simulink model "smm_with_grf_tilting_2d"  (R2014b)
settings: Solver=FixedStepDiscrete  StartTime=0.0  StopTime=inf  FixedStep=sample_time  RelTol=1e-3
undefined symbols (not defined in the file or in its folder): A_kalman_fourbar_gear, A_kalman_transverse, A_kalman_vertical, A_lpf_dtau, A_lpf_leg_spring, alpha_apex, B1_lpf_dtau, B1_lpf_leg_spring, B2_lpf_dtau, B2_lpf_leg_spring, B_kalman_fourbar_gear, B_kalman_transverse, B_kalman_vertical, b_virtual, boom_mount_angle, c_energy, C_kalman_fourbar_gear, C_kalman_transverse, C_kalman_vertical, com_leg_motor, com_torso, contact_threshold, control_start_time, d_vertical_boom_com_offset, d_vertical_com, d_y_com, desired_com_apex_height, desired_com_forward_velocity, desired_torso_angle, Discrete, fcut_contact, g, h_boom, HIP_MTR_MAX_CONT_TORQUE, i_robot, initial_dx_estimate, initial_dy_estimate, initial_dz_estimate, initial_z_estimate, j_leg, j_motor, j_rotor, j_segments, k0_virtual, k_placement, k_sea, kalman_load_to_deflect_transmission, kalman_stance_slip_threshold, kd_lateral, kd_motor, kd_torso, kp_lateral, kp_motor, kp_torso, l0_leg, l0_virtual, l_boom_projected, l_retract_delta, l_retract_swing_max, l_retract_swing_min ... (+59)
libraries: simulink x25, ctrlSharedLib x7, simulink_extras x1
(part 2 of 4)

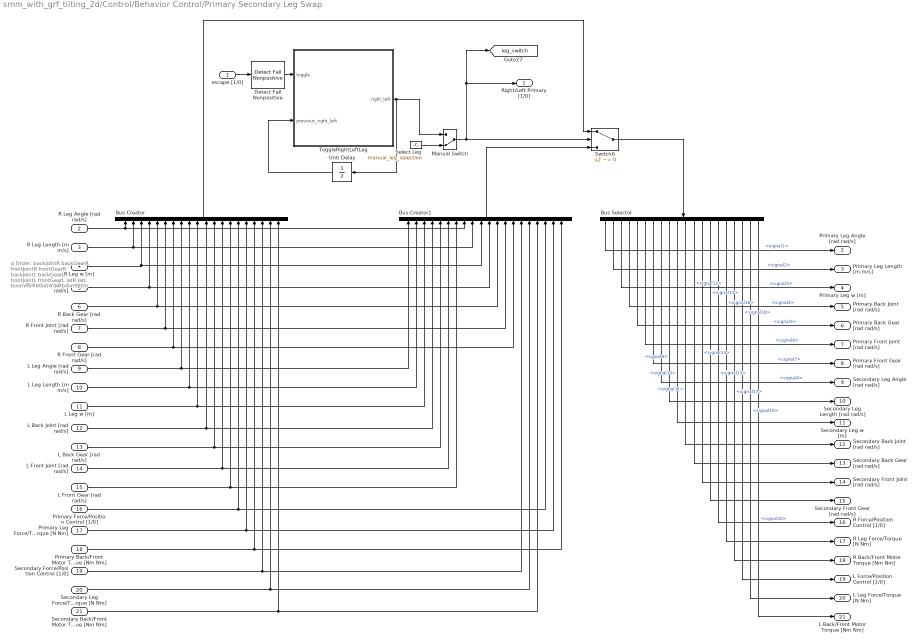
== system smm_with_grf_tilting_2d/Control/Behavior Control/Primary Secondary Leg Swap ==
  note: q Order:
      |
      | backJointR
      | backGearR
      | frontJointR
      | frontGearR
      |
      | backJointL
      | backGearL
      | frontJointL
      | frontGearL
      |
      | latR
      | latL
      |
      | boomRoll
      | boomYaw
      | boomPitch
  escape [1/0] : Inport
  R Leg Angle [rad rad/s] : Inport  Port=2
  R Leg Length [m m/s] : Inport  Port=3
  R Leg w [m] : Inport  Port=4
  R Back Joint [rad rad/s] : Inport  Port=5
  R Back Gear [rad rad/s] : Inport  Port=6
  R Front Joint [rad rad/s] : Inport  Port=7
  R Front Gear [rad rad/s] : Inport  Port=8
  L Leg Angle [rad rad/s] : Inport  Port=9
  L Leg Length [m m/s] : Inport  Port=10
  L Leg w [m] : Inport  Port=11
  L Back Joint [rad rad/s] : Inport  Port=12
  L Back Gear [rad rad/s] : Inport  Port=13
  L Front Joint [rad rad/s] : Inport  Port=14
  L Front Gear [rad rad/s] : Inport  Port=15
  Primary Force/Position Control [1/0] : Inport  Port=16
  Primary Leg Force/Torque [N Nm] : Inport  Port=17
  Primary Back/Front Motor Torque [Nm Nm] : Inport  Port=18
  Secondary Force/Position Control [1/0] : Inport  Port=19
  Secondary Leg Force/Torque [N Nm] : Inport  Port=20
  Secondary Back/Front Motor Torque [Nm Nm] : Inport  Port=21
  Bus Creator : BusCreator  Inputs=20
  Bus Creator1 : BusCreator  Inputs=20
  Bus Selector : BusSelector  OutputSignals=signal1,signal2,signal3,signal4,signal5,signal6,signal7,signal8,signal9,signal10,signal11,signal12,signal13,signal14,signal15,signal16,signal17,signal18,signal19,signal20
  Detect Fall Nonpositive : simulink/Logic and Bit Operations/Detect Fall Nonpositive  vinit=0  InputProcessing=Inherited  OutDataTypeStr=boolean
  Manual Switch : ManualSwitch  CurrentSetting=0
  Select Leg : Constant  Value=manual_leg_selection  OutDataTypeStr=boolean
  Switch6 : Switch  Criteria=u2 ~= 0  OutDataTypeStr=Inherit: Inherit via back propagation  ZeroCross=off
  ToggleRightLeftLeg : MATLAB Function  TreatAsAtomicUnit=on
      settings: MinAlgLoopOccurrences=on
  Unit Delay : UnitDelay  InitialCondition=1  SampleTime=sample_time
  Right/Left Primary [1/0] : Outport
  Primary Leg Angle [rad rad/s] : Outport  Port=2
  Primary Leg Length [m m/s] : Outport  Port=3
  Primary Leg w [m] : Outport  Port=4
  Primary Back Joint [rad rad/s] : Outport  Port=5
  Primary Back Gear [rad rad/s] : Outport  Port=6
  Primary Front Joint [rad rad/s] : Outport  Port=7
  Primary Front Gear [rad rad/s] : Outport  Port=8
  Secondary Leg Angle [rad rad/s] : Outport  Port=9
  Secondary Leg Length [rad rad/s] : Outport  Port=10
  Secondary Leg w [m] : Outport  Port=11
  Secondary Back Joint [rad rad/s] : Outport  Port=12
  Secondary Back Gear [rad rad/s] : Outport  Port=13
  Secondary Front Joint [rad rad/s] : Outport  Port=14
  Secondary Front Gear [rad rad/s] : Outport  Port=15
  R Force/Position Control [1/0] : Outport  Port=16
  R Leg Force/Torque [N Nm] : Outport  Port=17
  R Back/Front Motor Torque [Nm Nm] : Outport  Port=18
  L Force/Position Control [1/0] : Outport  Port=19
  L Leg Force/Torque [N Nm] : Outport  Port=20
  L Back/Front Motor Torque [Nm Nm] : Outport  Port=21
  tag scope: leg_switch=global
  wires:
  Unit Delay/1 -> ToggleRightLeftLeg/2(previous_right_left)
  Detect Fall Nonpositive/1 -> ToggleRightLeftLeg/1(toggle)
  escape [1/0]/1 -> Detect Fall Nonpositive/1
  ToggleRightLeftLeg/1(right_left) -> Unit Delay/1, Manual Switch/1
  Manual Switch/1 -> [leg_switch], Right/Left Primary [1/0]/1, Switch6/2
  Select Leg/1 -> Manual Switch/2
  R Leg w [m]/1 -> Bus Creator1/10, Bus Creator/3
  R Leg Angle [rad rad/s]/1 -> Bus Creator1/8, Bus Creator/1
  R Leg Length [m m/s]/1 -> Bus Creator1/9, Bus Creator/2
  Bus Creator/1 -> Switch6/1
  Bus Creator1/1 -> Switch6/3
  R Back Joint [rad rad/s]/1 -> Bus Creator1/11, Bus Creator/4
  R Back Gear [rad rad/s]/1 -> Bus Creator1/12, Bus Creator/5
  R Front Joint [rad rad/s]/1 -> Bus Creator1/13, Bus Creator/6
  R Front Gear [rad rad/s]/1 -> Bus Creator1/14, Bus Creator/7
  L Leg Angle [rad rad/s]/1 -> Bus Creator1/1, Bus Creator/8
  L Leg Length [m m/s]/1 -> Bus Creator1/2, Bus Creator/9
  L Leg w [m]/1 -> Bus Creator1/3, Bus Creator/10
  L Back Joint [rad rad/s]/1 -> Bus Creator1/4, Bus Creator/11
  L Back Gear [rad rad/s]/1 -> Bus Creator1/5, Bus Creator/12
  L Front Joint [rad rad/s]/1 -> Bus Creator/13, Bus Creator1/6
  L Front Gear [rad rad/s]/1 -> Bus Creator1/7, Bus Creator/14
  Primary Force/Position Control [1/0]/1 -> Bus Creator1/18, Bus Creator/15
  Primary Leg Force/Torque [N Nm]/1 -> Bus Creator1/19, Bus Creator/16
  Primary Back/Front Motor Torque [Nm Nm]/1 -> Bus Creator1/20, Bus Creator/17
  Secondary Force/Position Control [1/0]/1 -> Bus Creator1/15, Bus Creator/18
  Secondary Leg Force/Torque [N Nm]/1 -> Bus Creator1/16, Bus Creator/19
  Secondary Back/Front Motor Torque [Nm Nm]/1 -> Bus Creator1/17, Bus Creator/20
  Switch6/1 -> Bus Selector/1
  Bus Selector/1 -> Primary Leg Angle [rad rad/s]/1  "<signal1>"
  Bus Selector/2 -> Primary Leg Length [m m/s]/1  "<signal2>"
  Bus Selector/3 -> Primary Leg w [m]/1  "<signal3>"
  Bus Selector/4 -> Primary Back Joint [rad rad/s]/1  "<signal4>"
  Bus Selector/5 -> Primary Back Gear [rad rad/s]/1  "<signal5>"
  Bus Selector/6 -> Primary Front Joint [rad rad/s]/1  "<signal6>"
  Bus Selector/7 -> Primary Front Gear [rad rad/s]/1  "<signal7>"
  Bus Selector/8 -> Secondary Leg Angle [rad rad/s]/1  "<signal8>"
  Bus Selector/9 -> Secondary Leg Length [rad rad/s]/1  "<signal9>"
  Bus Selector/10 -> Secondary Leg w [m]/1  "<signal10>"
  Bus Selector/11 -> Secondary Back Joint [rad rad/s]/1  "<signal11>"
  Bus Selector/12 -> Secondary Back Gear [rad rad/s]/1  "<signal12>"
  Bus Selector/13 -> Secondary Front Joint [rad rad/s]/1  "<signal13>"
  Bus Selector/14 -> Secondary Front Gear [rad rad/s]/1  "<signal14>"
  Bus Selector/15 -> R Force/Position Control [1/0]/1  "<signal15>"
  Bus Selector/16 -> R Leg Force/Torque [N Nm]/1  "<signal16>"
  Bus Selector/17 -> R Back/Front Motor Torque [Nm Nm]/1  "<signal17>"
  Bus Selector/18 -> L Force/Position Control [1/0]/1  "<signal18>"
  Bus Selector/19 -> L Leg Force/Torque [N Nm]/1  "<signal19>"
  Bus Selector/20 -> L Back/Front Motor Torque [Nm Nm]/1  "<signal20>"

== system smm_with_grf_tilting_2d/Control/Behavior Control/R Leg Calculator ==
  Front [rad rad/s] : Inport
  Back [rad rad/s] : Inport  Port=2
  Demux1 : Demux  Outputs=2
  Gain1 : Gain  Gain=2*l_seg
  Gain2 : Gain  Gain=l_seg
  Gain3 : Gain  Gain=-1
  Gain4 : Gain  Gain=0.5
  Gain5 : Gain  Gain=0.5
  Gain6 : Gain  Gain=2
  Mux1 : Mux  Inputs=2
  Product : Product  RndMeth=Zero
  Sum4 : Sum  Inputs=+|+
  Sum5 : Sum  Inputs=+|-
  Trigonometric Function : Trigonometry  Operator=cos
  Trigonometric Function1 : Trigonometry
  "Leg Length [m m/s] " : Outport
  Leg Angle [rad rad/s] : Outport  Port=2
  Leg Splay [rad rad/s] : Outport  Port=3
  w [m] : Outport  Port=4
  wires:
  Gain5/1 -> Leg Angle [rad rad/s]/1
  Sum4/1 -> Gain5/1
  Mux1/1 -> "Leg Length [m m/s] "/1
  Sum5/1 -> Demux1/1, Leg Splay [rad rad/s]/1
  Gain2/1 -> Gain6/1, Product/1
  Demux1/1 -> Gain4/1
  Gain3/1 -> Product/2
  Demux1/2 -> Gain3/1
  Back [rad rad/s]/1 -> Sum5/1, Sum4/1
  Front [rad rad/s]/1 -> Sum4/2, Sum5/2
  Product/1 -> Mux1/2
  Trigonometric Function1/1 -> Gain2/1
  Gain1/1 -> Mux1/1
  Trigonometric Function/1 -> Gain1/1
  Gain4/1 -> Trigonometric Function/1, Trigonometric Function1/1
  Gain6/1 -> w [m]/1

== system smm_with_grf_tilting_2d/Control/Behavior Control/Raibert Initiated ==
  Enable : EnablePort  StatesWhenEnabling=reset
  Constant : Constant
  Hopping? : Outport  InitialOutput=[0]
  wires:
  Constant/1 -> Hopping?/1

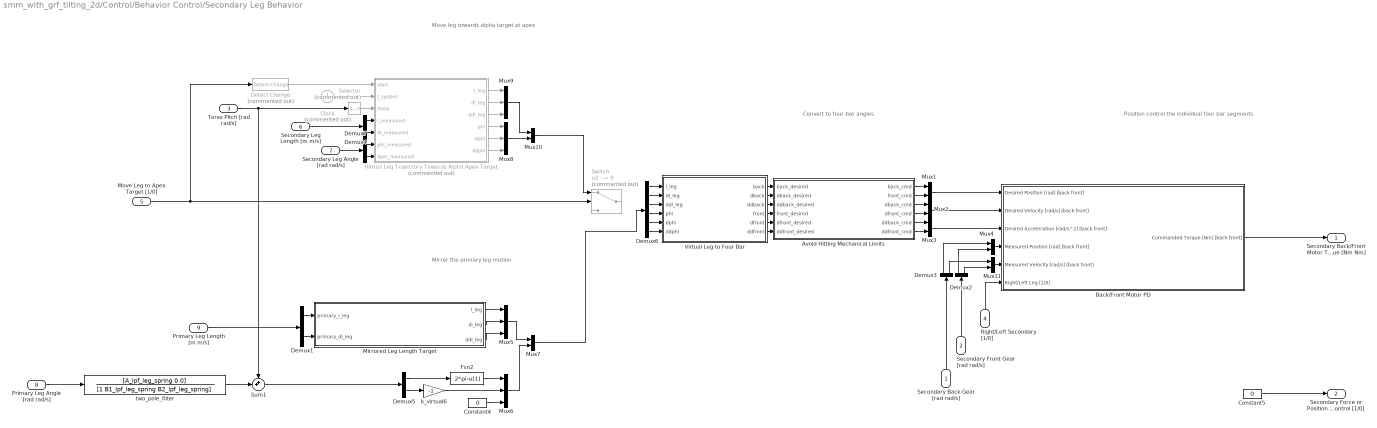
== system smm_with_grf_tilting_2d/Control/Behavior Control/Secondary Leg Behavior ==
  note: Mirror the primary
      | leg motion
  note: Move leg towards
      | alpha target at apex
  note: Position control the
      | individual four bar segments
  note: Convert to
      | four-bar angles
  Secondary Back Gear [rad rad/s] : Inport
  Secondary Front Gear [rad rad/s] : Inport  Port=2
  Torso Pitch [rad rad/s] : Inport  Port=3
  Right/Left Secondary [1/0] : Inport  Port=4
  Move Leg to Apex Target [1/0] : Inport  Port=5
  Secondary Leg Length [m m/s] : Inport  Port=6
  Secondary Leg Angle [rad rad/s] : Inport  Port=7
  Primary Leg Angle [rad rad/s] : Inport  Port=8
  Primary Leg Length [m m/s] : Inport  Port=9
  Avoid Hitting Mechanical Limits : MATLAB Function  TreatAsAtomicUnit=on
  Back/Front Motor PD : Subsystem
  Clock : Clock  Commented=on
  Constant4 : Constant  Value=0
  Constant5 : Constant  Value=0  OutDataTypeStr=boolean
  Demux{1..5,7} (6 alike) : Demux  Outputs=2
  Demux6 : Demux  Outputs=6
  Detect Change : simulink/Logic and Bit Operations/Detect Change  Commented=on  vinit=0  InputProcessing=Inherited  OutDataTypeStr=boolean
  Fcn2 : Fcn  Expr=2*pi-u(1)
  Mirrored Leg Length Target : MATLAB Function  TreatAsAtomicUnit=on
  Mux{1..4,7,10..11} (7 alike) : Mux  Inputs=2
  Mux{5..6,8..9} (4 alike) : Mux  Inputs=3
  Selector : Selector  Commented=on  InputPortWidth=2  Indices=[1]
  Sum1 : Sum  Inputs=++|
  Switch : Switch  Commented=on  Criteria=u2 ~= 0
  Virtual Leg Trajectory Towards Alpha Apex Target : MATLAB Function  Commented=on  TreatAsAtomicUnit=on
  Virtual Leg to Four Bar : MATLAB Function  TreatAsAtomicUnit=on
  k_virtual6 : Gain  Gain=-1
  two_pole_filter : DiscreteTransferFcn  Numerator=[A_lpf_leg_spring 0 0]  Denominator=[1 B1_lpf_leg_spring B2_lpf_leg_spring]  SampleTime=sample_time
  Secondary Back/Front Motor Torque [Nm Nm] : Outport
  Secondary Force or Position Control [1/0] : Outport  Port=2
  wires:
  Constant5/1 -> Secondary Force or Position Control [1/0]/1
  Back/Front Motor PD/1(Commanded Torque [Nm] [back front]) -> Secondary Back/Front Motor Torque [Nm Nm]/1
  Demux5/2 -> k_virtual6/1
  Demux5/1 -> Fcn2/1
  Primary Leg Angle [rad rad/s]/1 -> two_pole_filter/1
  Mirrored Leg Length Target/2(dl_leg) -> Mux5/2
  Mirrored Leg Length Target/3(ddl_leg) -> Mux5/3
  Mirrored Leg Length Target/1(l_leg) -> Mux5/1
  Constant4/1 -> Mux6/3
  k_virtual6/1 -> Mux6/2
  Fcn2/1 -> Mux6/1
  Move Leg to Apex Target [1/0]/1 -> Detect Change/1, Switch/2
  Mux7/1 -> Demux6/1
  Mux9/1 -> Mux10/1
  Mux8/1 -> Mux10/2
  Mux10/1 -> Switch/1
  Torso Pitch [rad rad/s]/1 -> Selector/1, Sum1/1
  Selector/1 -> Virtual Leg Trajectory Towards Alpha Apex Target/3(theta)
  Mux5/1 -> Mux7/1
  Mux6/1 -> Mux7/2
  Virtual Leg Trajectory Towards Alpha Apex Target/6(ddphi) -> Mux8/3
  Virtual Leg Trajectory Towards Alpha Apex Target/5(dphi) -> Mux8/2
  Virtual Leg Trajectory Towards Alpha Apex Target/4(phi) -> Mux8/1
  Virtual Leg Trajectory Towards Alpha Apex Target/3(ddl_leg) -> Mux9/3
  Virtual Leg Trajectory Towards Alpha Apex Target/2(dl_leg) -> Mux9/2
  Virtual Leg Trajectory Towards Alpha Apex Target/1(l_leg) -> Mux9/1
  Detect Change/1 -> Virtual Leg Trajectory Towards Alpha Apex Target/1(start)
  Clock/1 -> Virtual Leg Trajectory Towards Alpha Apex Target/2(t_system)
  Demux4/2 -> Virtual Leg Trajectory Towards Alpha Apex Target/5(dl_measured)
  Demux4/1 -> Virtual Leg Trajectory Towards Alpha Apex Target/4(l_measured)
  Demux7/1 -> Virtual Leg Trajectory Towards Alpha Apex Target/6(phi_measured)
  Demux7/2 -> Virtual Leg Trajectory Towards Alpha Apex Target/7(dphi_measured)
  Secondary Leg Length [m m/s]/1 -> Demux4/1
  Secondary Leg Angle [rad rad/s]/1 -> Demux7/1
  Virtual Leg to Four Bar/1(back) -> Avoid Hitting Mechanical Limits/1(back_desired)
  Virtual Leg to Four Bar/2(dback) -> Avoid Hitting Mechanical Limits/2(dback_desired)
  Virtual Leg to Four Bar/3(ddback) -> Avoid Hitting Mechanical Limits/3(ddback_desired)
  Virtual Leg to Four Bar/4(front) -> Avoid Hitting Mechanical Limits/4(front_desired)
  Virtual Leg to Four Bar/5(dfront) -> Avoid Hitting Mechanical Limits/5(dfront_desired)
  Virtual Leg to Four Bar/6(ddfront) -> Avoid Hitting Mechanical Limits/6(ddfront_desired)
  Demux6/1 -> Virtual Leg to Four Bar/1(l_leg)
  Demux6/2 -> Virtual Leg to Four Bar/2(dl_leg)
  Demux6/3 -> Virtual Leg to Four Bar/3(ddl_leg)
  Demux6/4 -> Virtual Leg to Four Bar/4(phi)
  Demux6/5 -> Virtual Leg to Four Bar/5(dphi)
  Demux6/6 -> Virtual Leg to Four Bar/6(ddphi)
  Mux11/1 -> Back/Front Motor PD/5(Measured Velocity [rad/s] [back front])
  Demux2/2 -> Mux11/2
  Mux4/1 -> Back/Front Motor PD/4(Measured Position [rad] [back front])
  Mux1/1 -> Back/Front Motor PD/1(Desired Position [rad] [back front])
  Right/Left Secondary [1/0]/1 -> Back/Front Motor PD/6(Right/Left Leg [1/0])
  Demux3/2 -> Mux11/1
  Demux3/1 -> Mux4/1
  Avoid Hitting Mechanical Limits/2(front_cmd) -> Mux1/2
  Avoid Hitting Mechanical Limits/1(back_cmd) -> Mux1/1
  Demux2/1 -> Mux4/2
  Secondary Front Gear [rad rad/s]/1 -> Demux2/1
  Secondary Back Gear [rad rad/s]/1 -> Demux3/1
  Avoid Hitting Mechanical Limits/3(dback_cmd) -> Mux2/1
  Avoid Hitting Mechanical Limits/4(dfront_cmd) -> Mux2/2
  Avoid Hitting Mechanical Limits/5(ddback_cmd) -> Mux3/1
  Avoid Hitting Mechanical Limits/6(ddfront_cmd) -> Mux3/2
  Mux2/1 -> Back/Front Motor PD/2(Desired Velocity [rad/s] [back front])
  Mux3/1 -> Back/Front Motor PD/3(Desired Acceleration [rad/s^2] [back front])
  two_pole_filter/1 -> Sum1/2
  Sum1/1 -> Demux5/1
  Demux1/1 -> Mirrored Leg Length Target/1(primary_l_leg)
  Demux1/2 -> Mirrored Leg Length Target/2(primary_dl_leg)
  Primary Leg Length [m m/s]/1 -> Demux1/1

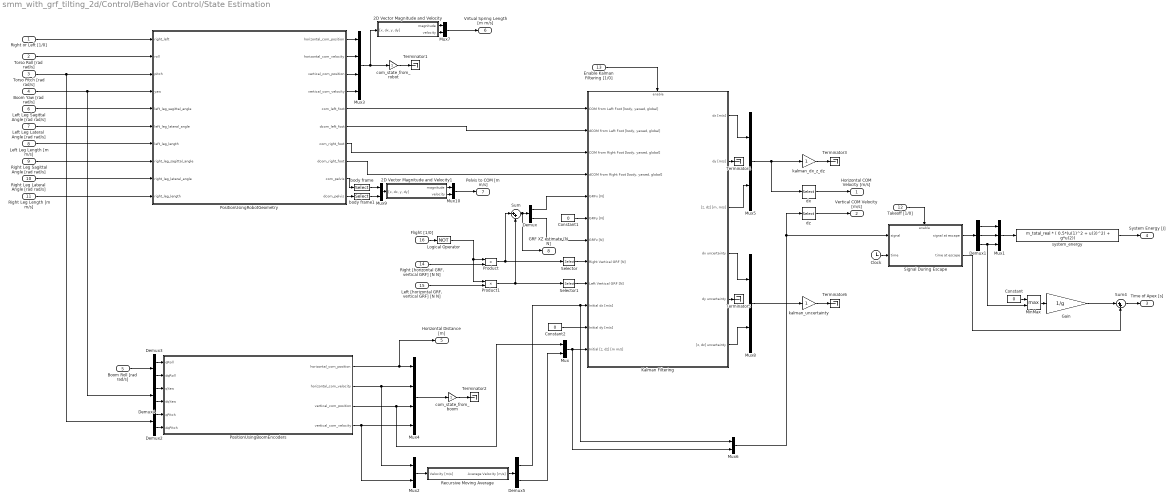
== system smm_with_grf_tilting_2d/Control/Behavior Control/State Estimation ==
  Right or Left [1/0] : Inport
  Torso Roll [rad rad/s] : Inport  Port=2
  Torso Pitch [rad rad/s] : Inport  Port=3
  Boom Yaw [rad rad/s] : Inport  Port=4
  Boom Roll [rad rad/s] : Inport  Port=5
  Left Leg Sagittal Angle [rad rad/s] : Inport  Port=6
  Left Leg Lateral  Angle [rad rad/s] : Inport  Port=7
  Left Leg Length [m m/s] : Inport  Port=8
  Right Leg Sagittal Angle [rad rad/s] : Inport  Port=9
  Right Leg Lateral  Angle [rad rad/s] : Inport  Port=10
  Right Leg Length [m m/s] : Inport  Port=11
  Takeoff [1/0] : Inport  Port=12
  Enable Kalman Filtering [1/0] : Inport  Port=13
  "Right [horizontal GRF, vertical GRF] [N N]" : Inport  Port=14
  "Left [horizontal GRF, vertical GRF] [N N]" : Inport  Port=15
  Flight [1/0] : Inport  Port=16
  2D Vector Magnitude and Velocity : Subsystem
  2D Vector Magnitude and Velocity1 : Subsystem
  Clock : Clock
  Constant : Constant  Value=0
  Constant1 : Constant  Value=0
  Constant2 : Constant  Value=0
  Demux{,2..5} (5 alike) : Demux  Outputs=2
  Demux1 : Demux  Outputs=3
  Gain : Gain  Gain=1/g
  Kalman Filtering : Subsystem
  Logical Operator : Logic  Operator=NOT  AllPortsSameDT=off  OutDataTypeStr=boolean
  MinMax : MinMax  Function=max  Inputs=2
  Mux{,2,5..10} (8 alike) : Mux  Inputs=2
  Mux1 : Mux  Inputs=3
  Mux3 : Mux
  Mux4 : Mux
  PositionUsingBoomEncoders : MATLAB Function  TreatAsAtomicUnit=on
  PositionUsingRobotGeometry : MATLAB Function  TreatAsAtomicUnit=on
  Product : Product
  Product1 : Product
  Recursive Moving Average : Subsystem
  Selector : Selector  InputPortWidth=2  Indices=[2]
  Selector1 : Selector  InputPortWidth=2  Indices=[2]
  Signal During Escape : Subsystem
  Sum : Sum  Inputs=|++
  Sum4 : Sum  Inputs=|++
  Terminator{1..6} (6 alike) : Terminator
  body frame : Selector  InputPortWidth=9  Indices=[1 3]
  body frame1 : Selector  InputPortWidth=9  Indices=[1 3]
  com_state_from_boom : Gain
  com_state_from_robot : Gain
  dx : Selector  InputPortWidth=3  Indices=[1]
  dz : Selector  InputPortWidth=3  Indices=[3]
  kalman_dx_z_dz : Gain
  kalman_uncertainty : Gain
  system_energy : Fcn  Expr=m_total_real * ( 0.5*(u(1)^2 + u(3)^2) + g*u(2))
  Horizontal COM Velocity [m/s] : Outport
  Vertical COM Velocity [m/s] : Outport  Port=2
  Time of Apex [s] : Outport  Port=3
  System Energy [J] : Outport  Port=4
  Horizontal Distance [m] : Outport  Port=5
  Virtual Spring Length [m m/s] : Outport  Port=6
  Pelvis to COM [m m/s] : Outport  Port=7
  GRF XZ estimate [N N] : Outport  Port=8
  wires:
  Gain/1 -> Sum4/1
  com_state_from_boom/1 -> Terminator2/1
  system_energy/1 -> System Energy [J]/1
  Clock/1 -> Signal During Escape/2(time)
  Demux1/3 -> MinMax/2, Mux1/3
  Signal During Escape/2(time at escape) -> Sum4/2
  Takeoff [1/0]/1 -> Signal During Escape/Enable
  Mux1/1 -> system_energy/1
  Demux1/1 -> Mux1/1
  Demux1/2 -> Mux1/2
  Sum4/1 -> Time of Apex [s]/1
  Kalman Filtering/1(dx [m/s]) -> Mux5/1
  MinMax/1 -> Gain/1
  Constant/1 -> MinMax/1
  Demux2/1 -> PositionUsingBoomEncoders/5(qPitch)
  Demux2/2 -> PositionUsingBoomEncoders/6(dqPitch)
  Mux3/1 -> 2D Vector Magnitude and Velocity/1("[x, dx, y, dy]"), com_state_from_robot/1
  com_state_from_robot/1 -> Terminator1/1
  PositionUsingRobotGeometry/4(vertical_com_velocity) -> Mux3/4
  PositionUsingRobotGeometry/3(vertical_com_position) -> Mux3/3
  PositionUsingRobotGeometry/2(horizontal_com_velocity) -> Mux3/2
  PositionUsingRobotGeometry/1(horizontal_com_position) -> Mux3/1
  PositionUsingBoomEncoders/1(horizontal_com_position) -> Horizontal Distance [m]/1, Mux4/1
  PositionUsingBoomEncoders/3(vertical_com_position) -> Mux/1, Mux4/3
  PositionUsingBoomEncoders/4(vertical_com_velocity) -> Mux2/2, Mux4/4
  Mux4/1 -> com_state_from_boom/1
  Left Leg Sagittal Angle [rad rad/s]/1 -> PositionUsingRobotGeometry/5(left_leg_sagittal_angle)
  Left Leg Lateral  Angle [rad rad/s]/1 -> PositionUsingRobotGeometry/6(left_leg_lateral_angle)
  Left Leg Length [m m/s]/1 -> PositionUsingRobotGeometry/7(left_leg_length)
  Right Leg Sagittal Angle [rad rad/s]/1 -> PositionUsingRobotGeometry/8(right_leg_sagittal_angle)
  Right Leg Lateral  Angle [rad rad/s]/1 -> PositionUsingRobotGeometry/9(right_leg_lateral_angle)
  Right Leg Length [m m/s]/1 -> PositionUsingRobotGeometry/10(right_leg_length)
  Right or Left [1/0]/1 -> PositionUsingRobotGeometry/1(right_left)
  Torso Roll [rad rad/s]/1 -> PositionUsingRobotGeometry/2(roll)
  Boom Yaw [rad rad/s]/1 -> PositionUsingRobotGeometry/4(yaw), Demux4/1
  Torso Pitch [rad rad/s]/1 -> PositionUsingRobotGeometry/3(pitch), Demux2/1
  Demux3/2 -> PositionUsingBoomEncoders/2(dqRoll)
  Demux3/1 -> PositionUsingBoomEncoders/1(qRoll)
  Boom Roll [rad rad/s]/1 -> Demux3/1
  Demux4/1 -> PositionUsingBoomEncoders/3(qYaw)
  Demux4/2 -> PositionUsingBoomEncoders/4(dqYaw)
  PositionUsingRobotGeometry/5(com_left_foot) -> Kalman Filtering/1("COM from Left Foot [body, yawed, global]")
  PositionUsingRobotGeometry/6(dcom_left_foot) -> Kalman Filtering/2("dCOM from Left Foot [body, yawed, global]")
  PositionUsingRobotGeometry/7(com_right_foot) -> Kalman Filtering/3("COM from Right Foot [body, yawed, global]")
  PositionUsingRobotGeometry/8(dcom_right_foot) -> Kalman Filtering/4("dCOM from Right Foot [body, yawed, global]")
  Kalman Filtering/2(dy [m/s]) -> Terminator4/1
  Kalman Filtering/3("[z, dz] [m, m/s]") -> Mux5/2
  Signal During Escape/1(signal at escape) -> Demux1/1
  Mux2/1 -> Recursive Moving Average/1(Velocity [m/s])
  dx/1 -> Horizontal COM Velocity [m/s]/1
  Mux6/1 -> Signal During Escape/1(signal), dz/1
  dz/1 -> Vertical COM Velocity [m/s]/1
  Constant1/1 -> Kalman Filtering/6(GRFy [N])
  Recursive Moving Average/1(Average Velocity [m/s]) -> Demux5/1
  Mux/1 -> Mux6/2, Kalman Filtering/12("Initial [z, dz] [m m/s]")
  Demux5/2 -> Mux/2
  Constant2/1 -> Kalman Filtering/11(Initial dy [m/s])
  PositionUsingBoomEncoders/2(horizontal_com_velocity) -> Mux2/1, Mux4/2
  Selector/1 -> Kalman Filtering/8(Right Vertical GRF [N])
  Selector1/1 -> Kalman Filtering/9(Left Vertical GRF [N])
  Product1/1 -> Sum/2, Selector1/1
  Product/1 -> Sum/1, Selector/1
  Sum/1 -> GRF XZ estimate [N N]/1, Demux/1
  Enable Kalman Filtering [1/0]/1 -> Kalman Filtering/Enable
  kalman_dx_z_dz/1 -> Terminator3/1
  Mux5/1 -> dx/1, kalman_dx_z_dz/1
  Demux5/1 -> Mux6/1, Kalman Filtering/10(Initial dx [m/s])
  Mux7/1 -> Virtual Spring Length [m m/s]/1
  Demux/1 -> Kalman Filtering/5(GRFx [N])
  Demux/2 -> Kalman Filtering/7(GRFz [N])
  Flight [1/0]/1 -> Logical Operator/1
  "Right [horizontal GRF, vertical GRF] [N N]"/1 -> Product/2
  Logical Operator/1 -> Product1/1, Product/1
  "Left [horizontal GRF, vertical GRF] [N N]"/1 -> Product1/2
  Kalman Filtering/4(dx uncertainty) -> Mux8/1
  Kalman Filtering/6("[z, dz] uncertainty") -> Mux8/2
  Kalman Filtering/5(dy uncertainty) -> Terminator5/1
  kalman_uncertainty/1 -> Terminator6/1
  Mux8/1 -> kalman_uncertainty/1
  PositionUsingRobotGeometry/10(dcom_pelvis) -> body frame1/1
  PositionUsingRobotGeometry/9(com_pelvis) -> body frame/1
  body frame/1 -> Mux9/1
  body frame1/1 -> Mux9/2
  Mux9/1 -> 2D Vector Magnitude and Velocity1/1("[x, dx, y, dy]")
  2D Vector Magnitude and Velocity/1(magnitude) -> Mux7/1
  2D Vector Magnitude and Velocity/2(velocity) -> Mux7/2
  2D Vector Magnitude and Velocity1/1(magnitude) -> Mux10/1
  2D Vector Magnitude and Velocity1/2(velocity) -> Mux10/2
  Mux10/1 -> Pelvis to COM [m m/s]/1

== system smm_with_grf_tilting_2d/Control/Behavior Control/Torque Distribution Left ==
  Leg Torque [Nm] : Inport
  Leg Force [N] : Inport  Port=2
  w [m] : Inport  Port=3
  Gain : Gain  Gain=0.5
  Gain1 : Gain  Gain=0.5
  Motor Torque Saturation Optimization : MATLAB Function  TreatAsAtomicUnit=on
  Product : Product  RndMeth=Zero
  Sum : Sum  Inputs=|++
  Sum1 : Sum  Inputs=+-|
  Back Torque [Nm] : Outport
  Front Torque [Nm] : Outport  Port=2
  wires:
  Gain/1 -> Motor Torque Saturation Optimization/1(x1s)
  Gain1/1 -> Motor Torque Saturation Optimization/2(x2s)
  Product/1 -> Gain1/1
  Leg Force [N]/1 -> Product/1
  Motor Torque Saturation Optimization/2(t2) -> Sum/2, Sum1/2
  w [m]/1 -> Product/2
  Motor Torque Saturation Optimization/1(t1) -> Sum1/1, Sum/1
  Sum/1 -> Front Torque [Nm]/1
  Leg Torque [Nm]/1 -> Gain/1
  Sum1/1 -> Back Torque [Nm]/1

== system smm_with_grf_tilting_2d/Control/Behavior Control/Torque Distribution Right ==
  Leg Torque [Nm] : Inport
  Leg Force [N] : Inport  Port=2
  w [m] : Inport  Port=3
  Gain : Gain  Gain=0.5
  Gain1 : Gain  Gain=0.5
  Motor Torque Saturation Optimization : MATLAB Function  TreatAsAtomicUnit=on
  Product : Product  RndMeth=Zero
  Sum : Sum  Inputs=|++
  Sum1 : Sum  Inputs=+-|
  Back Torque [Nm] : Outport
  Front Torque [Nm] : Outport  Port=2
  wires:
  Sum1/1 -> Back Torque [Nm]/1
  Leg Torque [Nm]/1 -> Gain/1
  Sum/1 -> Front Torque [Nm]/1
  Motor Torque Saturation Optimization/1(t1) -> Sum/1, Sum1/1
  w [m]/1 -> Product/2
  Motor Torque Saturation Optimization/2(t2) -> Sum1/2, Sum/2
  Leg Force [N]/1 -> Product/1
  Product/1 -> Gain1/1
  Gain1/1 -> Motor Torque Saturation Optimization/2(x2s)
  Gain/1 -> Motor Torque Saturation Optimization/1(x1s)

== system smm_with_grf_tilting_2d/Control/Behavior Control/Virtual Spring Calculator ==
  "Stance Leg Angle [rad rad/s] " : Inport
  Stance Leg Length [m m/s] : Inport  Port=2
  Torso Angle [rad rad/s] : Inport  Port=3
  Demux : Demux  Outputs=2
  Demux1 : Demux  Outputs=2
  Demux2 : Demux  Outputs=2
  Mux3 : Mux  Inputs=2
  Mux4 : Mux  Inputs=2
  Virtual Spring Calculations : MATLAB Function  TreatAsAtomicUnit=on
  Spring Length [m m/s] : Outport
  Spring Alpha [rad rad/s] : Outport  Port=2  OutDataTypeStr=double  PortDimensions=2
  wires:
  Stance Leg Length [m m/s]/1 -> Demux1/1
  Mux3/1 -> Spring Length [m m/s]/1
  "Stance Leg Angle [rad rad/s] "/1 -> Demux2/1
  Torso Angle [rad rad/s]/1 -> Demux/1
  Demux/1 -> Virtual Spring Calculations/1(th)
  Demux/2 -> Virtual Spring Calculations/2(dth)
  Demux1/1 -> Virtual Spring Calculations/3(l)
  Demux2/1 -> Virtual Spring Calculations/5(phi)
  Demux2/2 -> Virtual Spring Calculations/6(dphi)
  Demux1/2 -> Virtual Spring Calculations/4(dl)
  Virtual Spring Calculations/1(alpha_v) -> Mux4/1
  Virtual Spring Calculations/2(dalpha_v) -> Mux4/2
  Virtual Spring Calculations/3(l_v) -> Mux3/1
  Virtual Spring Calculations/4(dl_v) -> Mux3/2
  Mux4/1 -> Spring Alpha [rad rad/s]/1

== system smm_with_grf_tilting_2d/Control/Behavior Control/dtau_des ==
  x : Inport
  Gain1 : Gain  Gain=1/sample_time
  difference : simulink/Discrete/Difference  ICPrevInput=0.0  InputProcessing=Inherited  OutMin=[]  OutMax=[]  OutDataType=fixdt(1, 16)  OutScaling=2^-10  DoSatur=off
  two_pole_filter : DiscreteTransferFcn  Numerator=[A_lpf_dtau 0 0]  Denominator=[1 B1_lpf_dtau B2_lpf_dtau]  SampleTime=sample_time
  dx/dt : Outport
  wires:
  two_pole_filter/1 -> dx/dt/1
  x/1 -> Gain1/1
  difference/1 -> two_pole_filter/1
  Gain1/1 -> difference/1

== system smm_with_grf_tilting_2d/Control/Behavior Control/Force Estimation/Contact Time ==
  Enable : EnablePort  StatesWhenEnabling=reset  ShowOutputPort=on
  Constant : Constant
  Discrete-Time Integrator : DiscreteIntegrator  IntegratorMethod=Accumulation: Forward Euler  gainval=sample_time  ExternalReset=rising  SampleTime=sample_time
  ts [s] : Outport  InitialOutput=[0]
  wires:
  Discrete-Time Integrator/1 -> ts [s]/1
  Enable/1 -> Discrete-Time Integrator/2
  Constant/1 -> Discrete-Time Integrator/1

== system smm_with_grf_tilting_2d/Control/Behavior Control/Force Estimation/Horizontal GRF ==
  Axial Force [N] : Inport
  Orthogonal Force [N] : Inport  Port=2
  Torso Pitch [rad] : Inport  Port=3
  Leg Angle [rad] : Inport  Port=4
  Gain : Gain  Gain=-1
  Product : Product
  Product1 : Product
  Sum : Sum  Inputs=++|
  Sum1 : Sum  Inputs=+|+
  Trigonometric Function : Trigonometry
  Trigonometric Function1 : Trigonometry  Operator=cos
  Horizontal Force [N] : Outport
  wires:
  Product1/1 -> Gain/1
  Sum1/1 -> Horizontal Force [N]/1
  Trigonometric Function1/1 -> Product1/2
  Orthogonal Force [N]/1 -> Product1/1
  Axial Force [N]/1 -> Product/1
  Leg Angle [rad]/1 -> Sum/2
  Torso Pitch [rad]/1 -> Sum/1
  Trigonometric Function/1 -> Product/2
  Sum/1 -> Trigonometric Function/1, Trigonometric Function1/1
  Product/1 -> Sum1/1
  Gain/1 -> Sum1/2

== system smm_with_grf_tilting_2d/Control/Behavior Control/Force Estimation/Last Contact Time ==
  ts [s] : Inport
  Trigger : TriggerPort  TriggerType=falling  PortDimensions=1
  Ts [s] : Outport  InitialOutput=[0]
  wires:
  ts [s]/1 -> Ts [s]/1

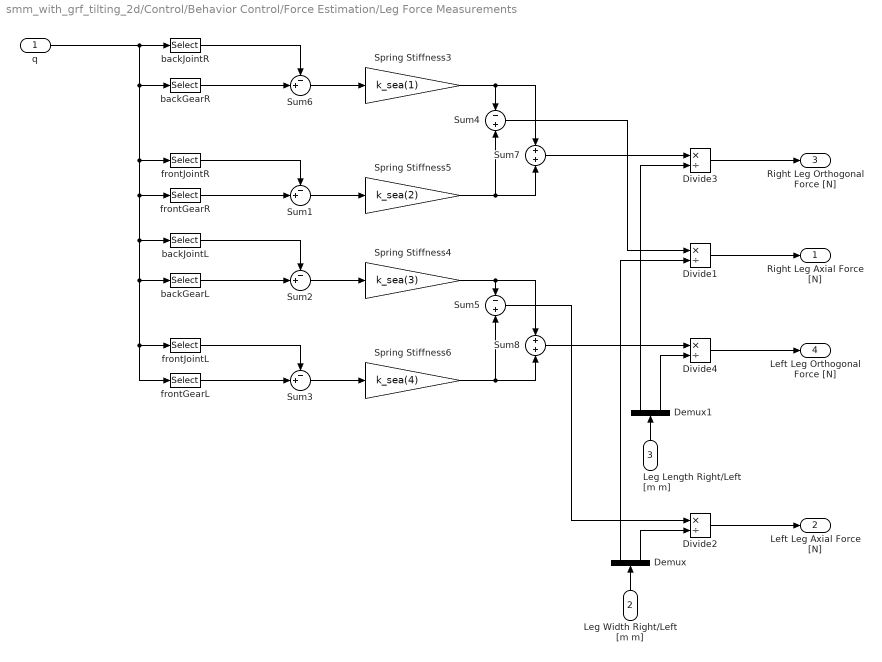
== system smm_with_grf_tilting_2d/Control/Behavior Control/Force Estimation/Leg Force Measurements ==
  q : Inport
  Leg Width Right/Left [m m] : Inport  Port=2
  Leg Length Right/Left [m m] : Inport  Port=3
  Demux : Demux  Outputs=2
  Demux1 : Demux  Outputs=2
  Divide{1..4} (4 alike) : Product  Inputs=*/
  Spring Stiffness3 : Gain  Gain=k_sea(1)
  Spring Stiffness4 : Gain  Gain=k_sea(3)
  Spring Stiffness5 : Gain  Gain=k_sea(2)
  Spring Stiffness6 : Gain  Gain=k_sea(4)
  Sum{1..3,6} (4 alike) : Sum  Inputs=-+|
  Sum4 : Sum  Inputs=-|+
  Sum5 : Sum  Inputs=-|+
  Sum7 : Sum  Inputs=+|+
  Sum8 : Sum  Inputs=+|+
  backGearL : Selector  InputPortWidth=13  Indices=[6]
  backGearR : Selector  InputPortWidth=13  Indices=[2]
  backJointL : Selector  InputPortWidth=13  Indices=[5]
  backJointR : Selector  InputPortWidth=13  Indices=[1]
  frontGearL : Selector  InputPortWidth=13  Indices=[8]
  frontGearR : Selector  InputPortWidth=13  Indices=[4]
  frontJointL : Selector  InputPortWidth=13  Indices=[7]
  frontJointR : Selector  InputPortWidth=13  Indices=[3]
  Right Leg Axial Force [N] : Outport
  Left Leg Axial Force [N] : Outport  Port=2
  Right Leg Orthogonal Force [N] : Outport  Port=3
  Left Leg Orthogonal Force [N] : Outport  Port=4
  wires:
  Sum3/1 -> Spring Stiffness6/1
  Sum2/1 -> Spring Stiffness4/1
  backJointL/1 -> Sum2/1
  frontGearL/1 -> Sum3/2
  frontJointL/1 -> Sum3/1
  backGearL/1 -> Sum2/2
  Sum6/1 -> Spring Stiffness3/1
  Sum1/1 -> Spring Stiffness5/1
  backJointR/1 -> Sum6/1
  frontGearR/1 -> Sum1/2
  frontJointR/1 -> Sum1/1
  backGearR/1 -> Sum6/2
  q/1 -> backGearR/1, backJointL/1, frontJointL/1, frontGearL/1, backGearL/1, frontGearR/1, frontJointR/1, backJointR/1
  Spring Stiffness3/1 -> Sum7/1, Sum4/1
  Spring Stiffness5/1 -> Sum7/2, Sum4/2
  Spring Stiffness6/1 -> Sum8/2, Sum5/2
  Sum4/1 -> Divide1/1
  Sum5/1 -> Divide2/1
  Leg Width Right/Left [m m]/1 -> Demux/1
  Demux/1 -> Divide1/2
  Demux/2 -> Divide2/2
  Divide1/1 -> Right Leg Axial Force [N]/1
  Divide2/1 -> Left Leg Axial Force [N]/1
  Spring Stiffness4/1 -> Sum8/1, Sum5/1
  Sum7/1 -> Divide3/1
  Sum8/1 -> Divide4/1
  Divide3/1 -> Right Leg Orthogonal Force [N]/1
  Divide4/1 -> Left Leg Orthogonal Force [N]/1
  Demux1/1 -> Divide3/2
  Demux1/2 -> Divide4/2
  Leg Length Right/Left [m m]/1 -> Demux1/1

== system smm_with_grf_tilting_2d/Control/Behavior Control/Force Estimation/Vertical GRF ==
  Axial Force [N] : Inport
  Orthogonal Force [N] : Inport  Port=2
  Torso Pitch [rad] : Inport  Port=3
  Leg Angle [rad] : Inport  Port=4
  Gain : Gain  Gain=-1
  Product : Product
  Product1 : Product
  Sum : Sum  Inputs=++|
  Sum1 : Sum  Inputs=+|+
  Trigonometric Function : Trigonometry  Operator=cos
  Trigonometric Function1 : Trigonometry
  Vertical Force [N] : Outport
  wires:
  Gain/1 -> Sum1/1
  Sum/1 -> Trigonometric Function1/1, Trigonometric Function/1
  Product/1 -> Gain/1
  Trigonometric Function/1 -> Product/2
  Torso Pitch [rad]/1 -> Sum/1
  Leg Angle [rad]/1 -> Sum/2
  Axial Force [N]/1 -> Product/1
  Orthogonal Force [N]/1 -> Product1/1
  Trigonometric Function1/1 -> Product1/2
  Sum1/1 -> Vertical Force [N]/1
  Product1/1 -> Sum1/2

== system smm_with_grf_tilting_2d/Control/Behavior Control/Primary Leg Behavior/Running ==
  note: Stance
  note: Flight
  Right/Left [1/0] : Inport
  Primary Leg Force [N] : Inport  Port=2
  Takeoff [1/0] : Inport  Port=3
  Flight [1/0] : Inport  Port=4
  Hopping [1/0] : Inport  Port=5
  Leg Length [m m/s] : Inport  Port=6
  Leg Angle [rad rad/s] : Inport  Port=7
  Torso Pitch [rad rad/s] : Inport  Port=8
  Stance Time [s] : Inport  Port=9
  dx [m/s] : Inport  Port=10
  Virtual Spring Length [m m/s] : Inport  Port=11
  Primary w [m] : Inport  Port=12
  Primary Back Gear [rad rad/s] : Inport  Port=13
  Primary Front Gear [rad rad/s] : Inport  Port=14
  Apex Time [s] : Inport  Port=15
  System Energy [J] : Inport  Port=16
  Horizontal Position [m] : Inport  Port=17
  Pelvis to COM [m m/s] : Inport  Port=18
  Flight : Subsystem
  Logical Operator1 : Logic  Operator=NOT  AllPortsSameDT=off  OutDataTypeStr=boolean
  Stance : Subsystem
  Leg Force Command (stance) [N] : Outport
  Leg Torque Command (stance) [Nm] : Outport  Port=2
  Back/Front Motor Torque (swing) [Nm Nm] : Outport  Port=3
  Primary Force or Position Control [1/0] : Outport  Port=4  OutDataTypeStr=boolean
  wires:
  System Energy [J]/1 -> Stance/1(System Energy [J])
  Leg Length [m m/s]/1 -> Stance/2(Leg Length [m m/s])
  Primary w [m]/1 -> Stance/4(Primary w [m])
  Virtual Spring Length [m m/s]/1 -> Stance/5(Virtual Spring Length [m m/s])
  Primary Leg Force [N]/1 -> Stance/6(Primary Leg Force [N])
  Stance/1(Leg Force Command (stance) [N]) -> Leg Force Command (stance) [N]/1
  Stance/2(Leg Torque Command (stance) [Nm]) -> Leg Torque Command (stance) [Nm]/1
  Torso Pitch [rad rad/s]/1 -> Flight/1(Torso Pitch [rad rad/s]), Stance/3(Torso Pitch [rad rad/s])
  Takeoff [1/0]/1 -> Flight/3(Takeoff [1/0])
  Hopping [1/0]/1 -> Stance/9(Hopping [1/0]), Flight/4(Hopping [1/0])
  Apex Time [s]/1 -> Flight/5(Apex Time [s])
  Stance Time [s]/1 -> Flight/7(Stance Time [s])
  dx [m/s]/1 -> Flight/8(dx [m/s])
  Horizontal Position [m]/1 -> Flight/9(Horizontal position [m])
  Right/Left [1/0]/1 -> Stance/10(Right/Left Primary [1/0]), Flight/10(Right/Left [1/0])
  Primary Back Gear [rad rad/s]/1 -> Flight/11(Primary Back Gear [rad rad/s])
  Primary Front Gear [rad rad/s]/1 -> Flight/12(Primary Front Gear [rad rad/s])
  Leg Angle [rad rad/s]/1 -> Flight/6(Leg Angle [rad rad/s]), Stance/8(Leg Angle [rad rad/s])
  Flight/1(Back/Front Motor Torque [Nm Nm]) -> Back/Front Motor Torque (swing) [Nm Nm]/1
  Logical Operator1/1 -> Primary Force or Position Control [1/0]/1, Stance/7(Stance [1/0])
  Flight [1/0]/1 -> Flight/2(Flight [1/0]), Logical Operator1/1
  Pelvis to COM [m m/s]/1 -> Flight/13(Pelvis to COM [m m/s])
  Flight/2(Desired Forward Velocity [m/s]) -> Stance/11(Desired Forward Velocity [m/s])

== system smm_with_grf_tilting_2d/Control/Behavior Control/Secondary Leg Behavior/Back//Front Motor PD ==
  Desired Position [rad] [back front] : Inport
  Desired Velocity [rad/s] [back front] : Inport  Port=2
  Desired Acceleration [rad/s^2] [back front] : Inport  Port=3
  Measured Position [rad] [back front] : Inport  Port=4
  Measured Velocity [rad/s] [back front] : Inport  Port=5
  Right/Left Leg [1/0] : Inport  Port=6
  Friction Compensation : Subsystem
  Product : Product
  Sum1 : Sum  Inputs=|++
  Sum2 : Sum  Inputs=|++
  Sum7 : Sum  Inputs=|+-
  Sum8 : Sum  Inputs=|+-
  Sum9 : Sum
  Switch : Switch  Criteria=u2 ~= 0
  kd : Gain  Gain=kd_motor
  kp : Gain  Gain=kp_motor
  left_inertias : Constant  Value=j_segments(3:4)
  reflected inertia : Constant  Value=j_motor
  right_inertias : Constant  Value=j_segments(1:2)
  Commanded Torque [Nm] [back front] : Outport
  wires:
  kp/1 -> Sum9/1
  Sum7/1 -> kp/1
  Measured Position [rad] [back front]/1 -> Sum7/2
  Sum9/1 -> Sum1/1
  Sum8/1 -> kd/1
  Desired Position [rad] [back front]/1 -> Sum7/1
  kd/1 -> Sum9/2
  Measured Velocity [rad/s] [back front]/1 -> Sum8/2
  Sum1/1 -> Sum2/1
  Desired Acceleration [rad/s^2] [back front]/1 -> Product/1
  Product/1 -> Sum1/2
  Right/Left Leg [1/0]/1 -> Friction Compensation/1(Right/Left [1/0]), Switch/2
  right_inertias/1 -> Switch/1
  left_inertias/1 -> Switch/3
  Sum2/1 -> Commanded Torque [Nm] [back front]/1
  Desired Velocity [rad/s] [back front]/1 -> Friction Compensation/2(Commanded Velocity [rad/s] [back front]), Sum8/1
  reflected inertia/1 -> Product/2

== system smm_with_grf_tilting_2d/Control/Behavior Control/State Estimation/2D Vector Magnitude and Velocity ==
  "[x, dx, y, dy]" : Inport
  Magnitude : Fcn  Expr=(u(1)^2 + u(3)^2)^(0.5)
  Velocity : Fcn  Expr=0.5*(2*u(1)*u(2) + 2*u(3)*u(4)) / (u(1)^2 + u(3)^2)^(0.5)
  magnitude : Outport
  velocity : Outport  Port=2
  wires:
  Magnitude/1 -> magnitude/1
  Velocity/1 -> velocity/1
  "[x, dx, y, dy]"/1 -> Magnitude/1, Velocity/1

== system smm_with_grf_tilting_2d/Control/Behavior Control/State Estimation/2D Vector Magnitude and Velocity1 ==
  "[x, dx, y, dy]" : Inport
  Magnitude : Fcn  Expr=(u(1)^2 + u(3)^2)^(0.5)
  Velocity : Fcn  Expr=0.5*(2*u(1)*u(2) + 2*u(3)*u(4)) / (u(1)^2 + u(3)^2)^(0.5)
  magnitude : Outport
  velocity : Outport  Port=2
  wires:
  "[x, dx, y, dy]"/1 -> Velocity/1, Magnitude/1
  Velocity/1 -> velocity/1
  Magnitude/1 -> magnitude/1

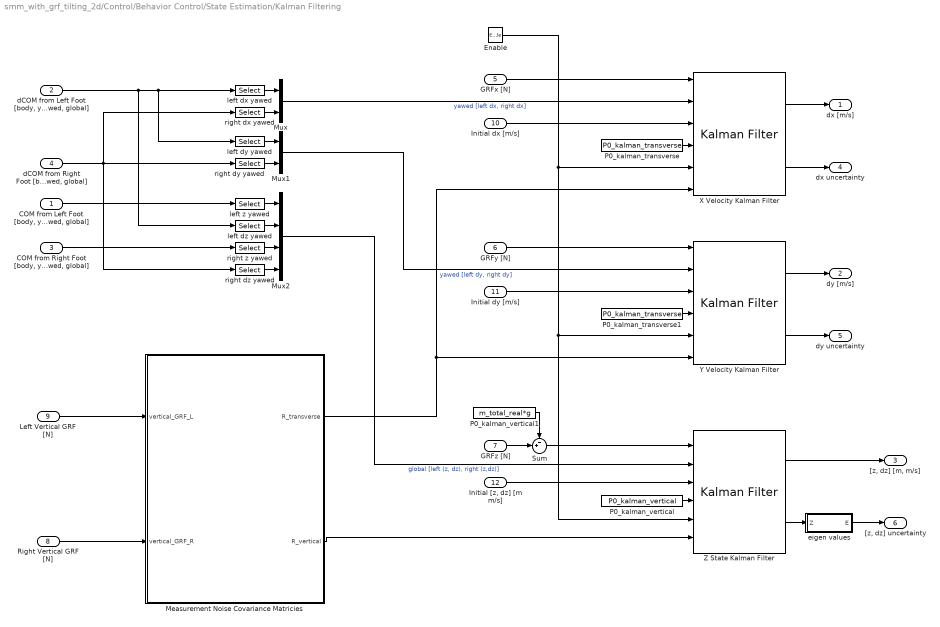
== system smm_with_grf_tilting_2d/Control/Behavior Control/State Estimation/Kalman Filtering ==
  "COM from Left Foot [body, yawed, global]" : Inport  SampleTime=sample_time
  "dCOM from Left Foot [body, yawed, global]" : Inport  Port=2  SampleTime=sample_time
  "COM from Right Foot [body, yawed, global]" : Inport  Port=3  SampleTime=sample_time
  "dCOM from Right Foot [body, yawed, global]" : Inport  Port=4  SampleTime=sample_time
  GRFx [N] : Inport  Port=5  SampleTime=sample_time
  GRFy [N] : Inport  Port=6  SampleTime=sample_time
  GRFz [N] : Inport  Port=7  SampleTime=sample_time
  Right Vertical GRF [N] : Inport  Port=8  SampleTime=sample_time
  Left Vertical GRF [N] : Inport  Port=9  SampleTime=sample_time
  Initial dx [m/s] : Inport  Port=10  PortDimensions=1  SampleTime=sample_time
  Initial dy [m/s] : Inport  Port=11  PortDimensions=1  SampleTime=sample_time
  "Initial [z, dz] [m m/s]" : Inport  Port=12  PortDimensions=2  SampleTime=sample_time
  Enable : EnablePort  ShowOutputPort=on
  Measurement Noise Covariance Matricies : MATLAB Function  TreatAsAtomicUnit=on
  Mux : Mux  Inputs=2
  Mux1 : Mux  Inputs=2
  Mux2 : Mux
  P0_kalman_transverse : Constant  Value=P0_kalman_transverse
  P0_kalman_transverse1 : Constant  Value=P0_kalman_transverse
  P0_kalman_vertical : Constant  Value=P0_kalman_vertical
  P0_kalman_vertical1 : Constant  Value=m_total_real*g
  Sum : Sum  Inputs=-+|
  X Velocity Kalman Filter : ctrlSharedLib/Kalman Filter  TimeDomain=Discrete-Time  UseCurrentEstimator=on  ModelSource=Individual A, B, C, D matrices  ModelSourceVariable=A_kf  A=A_kalman_transverse  B=B_kalman_transverse  C=C_kalman_transverse  D=0  NumberOfStates=2  NumberOfInputs=1  NumberOfOutputs=2  InitialEstimateSource=Input port  X0=initial_dx_estimate  P0=P0_kalman_transverse  UseK=off  UseGH=on  NumberOfProcessNoiseInputs=1  G=G_kalman_transverse  TimeInvariantG=on  H=0  TimeInvariantH=on  Q=Q_kalman_GRF  TimeInvariantQ=on  R=1  TimeInvariantR=off  N=0  TimeInvariantN=on  AddInputPort=on  AddEnablePort=off  ExternalReset=Either  OutputEstimatedY=off  OutputP=on  Ts=sample_time
  Y Velocity Kalman Filter : ctrlSharedLib/Kalman Filter  TimeDomain=Discrete-Time  UseCurrentEstimator=on  ModelSource=Individual A, B, C, D matrices  ModelSourceVariable=A_kf  A=A_kalman_transverse  B=B_kalman_transverse  C=C_kalman_transverse  D=0  NumberOfStates=2  NumberOfInputs=1  NumberOfOutputs=2  InitialEstimateSource=Input port  X0=initial_dy_estimate  P0=P0_kalman_transverse  UseK=off  UseGH=on  NumberOfProcessNoiseInputs=1  G=G_kalman_transverse  TimeInvariantG=on  H=0  TimeInvariantH=on  Q=Q_kalman_GRF  TimeInvariantQ=on  R=1  TimeInvariantR=off  N=0  TimeInvariantN=on  AddInputPort=on  AddEnablePort=off  ExternalReset=Either  OutputEstimatedY=off  OutputP=on  Ts=sample_time
  Z State Kalman Filter : ctrlSharedLib/Kalman Filter  TimeDomain=Discrete-Time  UseCurrentEstimator=on  ModelSource=Individual A, B, C, D matrices  ModelSourceVariable=A_kf  A=A_kalman_vertical  B=B_kalman_vertical  C=C_kalman_vertical  D=0  NumberOfStates=2  NumberOfInputs=1  NumberOfOutputs=2  InitialEstimateSource=Input port  X0=[initial_z_estimate; initial_dz_estimate]  P0=P0_kalman_vertical  UseK=off  UseGH=on  NumberOfProcessNoiseInputs=1  G=G_kalman_vertical  TimeInvariantG=on  H=0  TimeInvariantH=on  Q=Q_kalman_GRF  TimeInvariantQ=on  R=1  TimeInvariantR=off  N=0  TimeInvariantN=on  AddInputPort=on  AddEnablePort=off  ExternalReset=Either  OutputEstimatedY=off  OutputP=on  Ts=sample_time
  eigen values : MATLAB Function  TreatAsAtomicUnit=on
  left dx yawed : Selector  InputPortWidth=9  Indices=[4]
  left dy yawed : Selector  InputPortWidth=9  Indices=[5]
  left dz yawed : Selector  InputPortWidth=9  Indices=[6]
  left z yawed : Selector  InputPortWidth=9  Indices=[6]
  right dx yawed : Selector  InputPortWidth=9  Indices=[4]
  right dy yawed : Selector  InputPortWidth=9  Indices=[5]
  right dz yawed : Selector  InputPortWidth=9  Indices=[6]
  right z yawed : Selector  InputPortWidth=9  Indices=[6]
  dx [m/s] : Outport
  dy [m/s] : Outport  Port=2
  "[z, dz] [m, m/s]" : Outport  Port=3
  dx uncertainty : Outport  Port=4
  dy uncertainty : Outport  Port=5
  "[z, dz] uncertainty" : Outport  Port=6
  wires:
  GRFy [N]/1 -> Y Velocity Kalman Filter/1
  Mux2/1 -> Z State Kalman Filter/2  "global [left (z, dz), right (z,dz)]"
  GRFx [N]/1 -> X Velocity Kalman Filter/1
  Measurement Noise Covariance Matricies/2(R_vertical) -> Z State Kalman Filter/6
  Measurement Noise Covariance Matricies/1(R_transverse) -> X Velocity Kalman Filter/6, Y Velocity Kalman Filter/6
  Mux1/1 -> Y Velocity Kalman Filter/2  "yawed [left dy, right dy]"
  Sum/1 -> Z State Kalman Filter/1
  Mux/1 -> X Velocity Kalman Filter/2  "yawed [left dx, right dx]"
  Right Vertical GRF [N]/1 -> Measurement Noise Covariance Matricies/2(vertical_GRF_R)
  Left Vertical GRF [N]/1 -> Measurement Noise Covariance Matricies/1(vertical_GRF_L)
  Z State Kalman Filter/1 -> "[z, dz] [m, m/s]"/1
  Y Velocity Kalman Filter/1 -> dy [m/s]/1
  X Velocity Kalman Filter/1 -> dx [m/s]/1
  "dCOM from Left Foot [body, yawed, global]"/1 -> left dy yawed/1, left dx yawed/1, left dz yawed/1
  left dx yawed/1 -> Mux/1
  "dCOM from Right Foot [body, yawed, global]"/1 -> right dx yawed/1, right dz yawed/1, right dy yawed/1
  right dx yawed/1 -> Mux/2
  left dy yawed/1 -> Mux1/1
  right dy yawed/1 -> Mux1/2
  left z yawed/1 -> Mux2/1
  right z yawed/1 -> Mux2/3
  left dz yawed/1 -> Mux2/2
  right dz yawed/1 -> Mux2/4
  "COM from Left Foot [body, yawed, global]"/1 -> left z yawed/1
  "COM from Right Foot [body, yawed, global]"/1 -> right z yawed/1
  P0_kalman_transverse/1 -> X Velocity Kalman Filter/4
  Initial dx [m/s]/1 -> X Velocity Kalman Filter/3
  P0_kalman_transverse1/1 -> Y Velocity Kalman Filter/4
  Initial dy [m/s]/1 -> Y Velocity Kalman Filter/3
  P0_kalman_vertical/1 -> Z State Kalman Filter/4
  "Initial [z, dz] [m m/s]"/1 -> Z State Kalman Filter/3
  GRFz [N]/1 -> Sum/2
  P0_kalman_vertical1/1 -> Sum/1
  Enable/1 -> Z State Kalman Filter/5, Y Velocity Kalman Filter/5, X Velocity Kalman Filter/5
  X Velocity Kalman Filter/2 -> dx uncertainty/1
  Y Velocity Kalman Filter/2 -> dy uncertainty/1
  Z State Kalman Filter/2 -> eigen values/1(Z)
  eigen values/1(E) -> "[z, dz] uncertainty"/1

== system smm_with_grf_tilting_2d/Control/Behavior Control/State Estimation/Recursive Moving Average ==
  Velocity [m/s] : Inport
  Delay : Delay  DelayLength=velocity_avg_samples  InitialCondition=0  UseCircularBuffer=on  SampleTime=sample_time
  Gain : Gain  Gain=1/velocity_avg_samples
  Sum : Sum  Inputs=-++
  Unit Delay : UnitDelay  SampleTime=sample_time
  Average Velocity [m/s] : Outport
  wires:
  Unit Delay/1 -> Sum/3
  Gain/1 -> Average Velocity [m/s]/1
  Delay/1 -> Sum/1
  Sum/1 -> Gain/1, Unit Delay/1
  Velocity [m/s]/1 -> Sum/2, Delay/1

== system smm_with_grf_tilting_2d/Control/Behavior Control/State Estimation/Signal During Escape ==
  signal : Inport
  time : Inport  Port=2
  Enable : EnablePort
  signal at escape : Outport  InitialOutput=[0 0 desired_com_apex_height-0.1182]
  time at escape : Outport  Port=2  InitialOutput=[1]
  wires:
  time/1 -> time at escape/1
  signal/1 -> signal at escape/1
